simulink model "orologio_acuqa_simulink"  (R2022b)
settings: Solver=VariableStepAuto  StartTime=0.0  StopTime=50  RelTol=1e-3
values from neighbouring files (symbols this model uses):
  k1 = 3    [orologio_acqua_values.m]
  k2 = -1    [orologio_acqua_values.m]
  l0_1 = 10    [orologio_acqua_values.m]
  l0_2 = 5    [orologio_acqua_values.m]
  surface_tank1 = 12    [orologio_acqua_values.m]
  surface_tank2 = 5    [orologio_acqua_values.m]
undefined symbols (not defined in the file or in its folder): l0
settings Model: Creator=giuli  LastModifiedBy=giuli

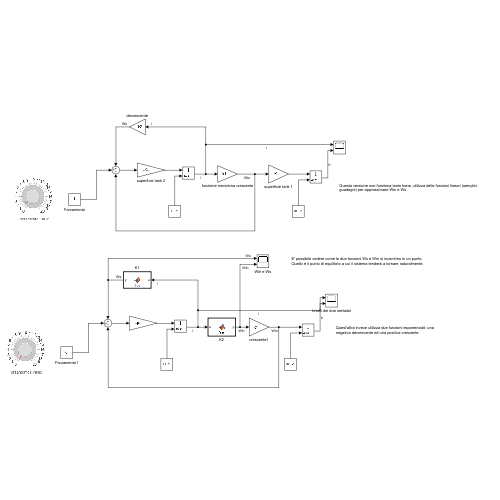
[thumbnail: Simulink's stored preview of the top-level diagram]
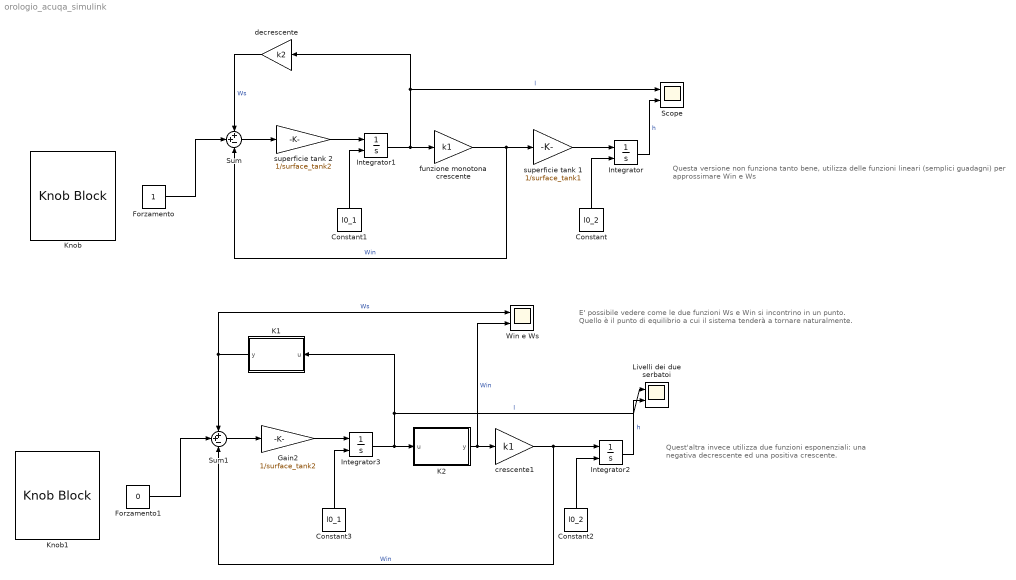
== system orologio_acuqa_simulink ==
  note: E' possibile vedere come le due funzioni Ws e Win si incontrino in un punto.
      | Quello è il punto di equilibrio a cui il sistema tenderà a tornare naturalmente.
  note: Quest'altra invece utilizza due funzioni esponenziali: una negativa decrescente ed una positiva crescente.
  note: Questa versione non funziona tanto bene, utilizza delle funzioni lineari (semplici guadagni) per approssimare Win e Ws
  Constant : Constant  Value=l0_2
  Constant1 : Constant  Value=l0_1
  Constant2 : Constant  Value=l0_2
  Constant3 : Constant  Value=l0_1
  Forzamento : Constant
  Forzamento1 : Constant  Value=0
  Gain2 : Gain  Gain=1/surface_tank2
  Integrator : Integrator  InitialConditionSource=external  InitialCondition=l0
  Integrator1 : Integrator  InitialConditionSource=external
  Integrator2 : Integrator  InitialConditionSource=external  InitialCondition=l0
  Integrator3 : Integrator  InitialConditionSource=external
  K1 : MATLAB Function  TreatAsAtomicUnit=on
  K2 : MATLAB Function  TreatAsAtomicUnit=on
  Knob : KnobBlock  LabelPosition=Bottom  ScaleMax=20  TickInterval=1
  Knob1 : KnobBlock  LabelPosition=Bottom  ScaleMax=20  TickInterval=1
  Livelli dei due serbatoi : Scope  NumInputPorts=2
  Scope : Scope  NumInputPorts=2
  Sum : Sum  Inputs=++-
  Sum1 : Sum  Inputs=++-
  Win e Ws : Scope  NumInputPorts=2
  crescente1 : Gain  Gain=k1
  decrescente : Gain  Gain=k2
  funzione monotona crescente : Gain  Gain=k1
  superficie tank 1 : Gain  Gain=1/surface_tank1
  superficie tank 2 : Gain  Gain=1/surface_tank2
  wires:
  Integrator1/1 -> decrescente/1, Scope/1, funzione monotona crescente/1  "l"
  Constant/1 -> Integrator/2
  Constant1/1 -> Integrator1/2
  superficie tank 2/1 -> Integrator1/1
  funzione monotona crescente/1 -> Sum/3, superficie tank 1/1  "Win"
  superficie tank 1/1 -> Integrator/1
  Sum/1 -> superficie tank 2/1
  decrescente/1 -> Sum/1  "Ws"
  Integrator/1 -> Scope/2  "h"
  Forzamento/1 -> Sum/2
  Forzamento1/1 -> Sum1/2
  Integrator2/1 -> Livelli dei due serbatoi/2  "h"
  Constant2/1 -> Integrator2/2
  Integrator3/1 -> K2/1(u), K1/1(u), Livelli dei due serbatoi/1  "l"
  Sum1/1 -> Gain2/1
  Constant3/1 -> Integrator3/2
  K2/1(y) -> Win e Ws/2, crescente1/1  "Win"
  crescente1/1 -> Sum1/3, Integrator2/1  "Win"
  Gain2/1 -> Integrator3/1
  K1/1(y) -> Win e Ws/1, Sum1/1  "Ws"

== matlab function orologio_acuqa_simulink/K2 ==
  data: u input; y output
function y = fcn(u)

y = 1-exp(-u);

== matlab function orologio_acuqa_simulink/K1 ==
  data: u input; y output
function y = fcn(u)

y = exp(-u);
